simulink model "board_testa"  (R2021b)
settings: Solver=FixedStepAuto  StartTime=0.0  StopTime=inf  RelTol=1e-3  EnableMultiTasking=on
undefined symbols (not defined in the file or in its folder): CR, LF
libraries: arduinolib x5, embeddedblockslib x1
settings Model: ExtModeTrigDuration=2  Creator=eduar  LastModifiedBy=ernesto
settings OptimizationCC: EnhancedBackFolding=on  PassReuseOutputArgsAs=Individual arguments  ZeroExternalMemoryAtStartup=off  ZeroInternalMemoryAtStartup=off  MaxStackSize=64  OptimizeBlockOrder=speed  DifferentSizesBufferReuse=on  OptimizationCustomize=off  EfficientTunableParamExpr=on
settings DebuggingCC: ParameterTunabilityLossMsg=error
settings HardwareCC: ProdBitPerPointer=32  ProdBitPerSizeT=32  ProdBitPerPtrDiffT=32  ProdLargestAtomicInteger=Long  ProdLargestAtomicFloat=Double  ProdWordSize=32  ProdHWDeviceType=ARM Compatible->ARM Cortex  UseEmbeddedCoderFeatures=off
settings SFSimCC: SimCustomHeaderCode="#include \"script\\callback.h\""  SimUserSources=script\callback.c  MATLABDynamicMemAlloc=off
settings RTWCC: Description=Embedded Coder  SystemTargetFile=ert.tlc  HardwareBoard=Arduino Due  TemplateMakefile=ert_default_tmf  RTWUseSimCustomCode=on  CustomHeaderCode="#include \"script\\callback.h\""  CustomSource=script\callback.c  Toolchain=Arduino ARM  BuildConfiguration=Faster Runs
settings CodeAppCC: ForceParamTrailComments=on  IgnoreCustomStorageClasses=off  OperatorAnnotations=on  SimulinkDataObjDesc=on  SFDataObjDesc=on  InsertBlockDesc=on
settings ERTTargetCC: SupportContinuousTime=on  SupportNonInlinedSFcns=on  SupportVariableSizeSignals=on  ExtModeTransport=3  ExtModeStaticAlloc=on  ExtModeStaticAllocSize=24576  ExtModeMexFile=ext_xcp  ExtModeIntrfLevel=Level2 - Open

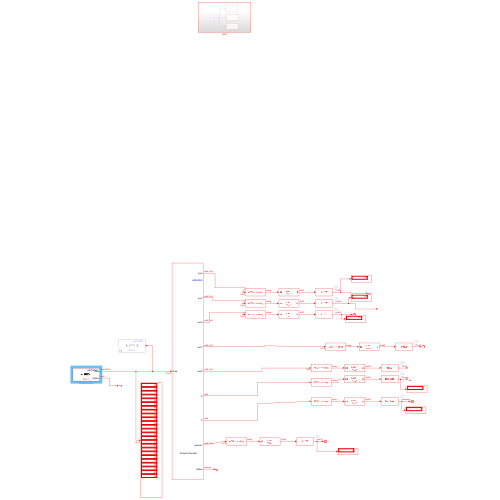
[thumbnail: Simulink's stored preview of the top-level diagram]
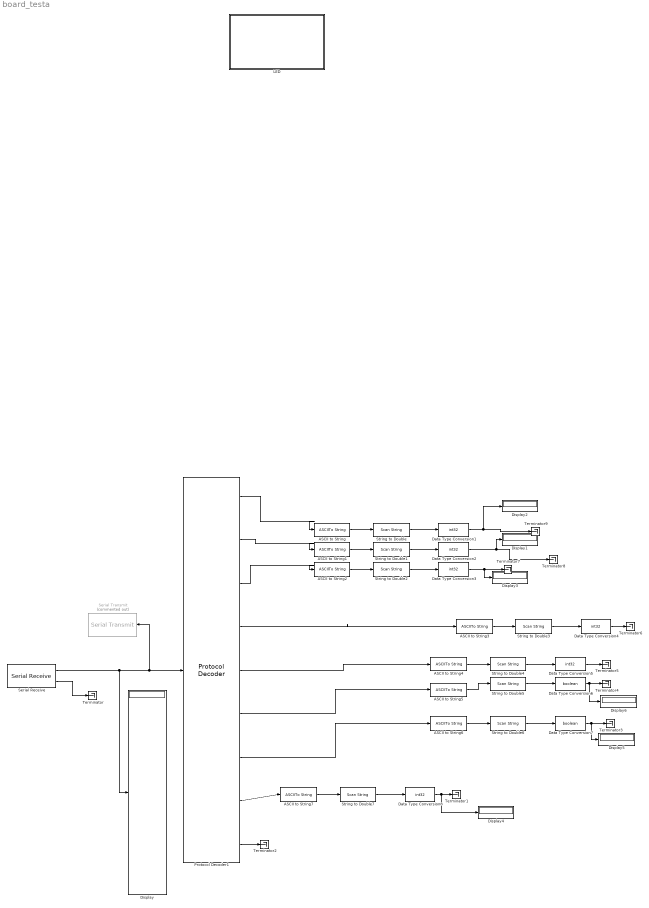
== system board_testa ==
  ASCII to String{,1..7} (8 alike) : ASCIIToString
  Data Type Conversion{1..5,8} (6 alike) : DataTypeConversion  OutDataTypeStr=int32  RndMeth=Round
  Data Type Conversion6 : DataTypeConversion  OutDataTypeStr=boolean  RndMeth=Round
  Data Type Conversion7 : DataTypeConversion  OutDataTypeStr=boolean  RndMeth=Round
  Display{,1..6} (7 alike) : Display
  LED : Subsystem
  Protocol Decoder1 : embeddedblockslib/Protocol Decoder  IsParseCSV=off  Header='@'  FieldTable={ 'joyX', '4', 'uint8', 'Little endian'; 'joyY', '4', 'uint8', 'Little endian'; 'accX', '4', 'uint8', 'Little endian'; 'accY', '4', 'uint8', 'Little endian'; 'accZ', '4', 'uint8', 'Little endian'; 'Z', '1', 'uint8', 'Little endian'; 'C', '1', 'uint8', 'Little endian'; 'remote1', '2', 'uint8', 'Little endian' }  IsVariableSizeLastField=off  MaxVariableSizeFieldLength=[]  IsChecksumRequired=off  ChecksumAlgorithm=XOR of bytes  ChecksumSize=[]  TerminatorOption=CR/LF ('\r\n')  CustomTerminatorVal=[]  IsInputLengthAvailable=off  Logo=ARDUINO
      settings: SourceProductBaseCode=ARDUINO,TIC2000
  Serial Receive : arduinolib/Serial Receive  isARMArch=on  portNumber=1  DataType=uint8  Datalength=25  SampleTime=0.01  showOutStatus=on  blockPlatform=arduino
      settings: SourceProductBaseCode=ARDUINO
  Serial Transmit : arduinolib/Serial Transmit  Commented=on  portNumber=0  sendmode=write  sendformat=Decimal  floatprecision=2  blockPlatform=arduino
  String to Double : ScanString  Format="\"%d\""
  String to Double1 : ScanString  Format="\"%d\""
  String to Double2 : ScanString  Format="\"%d\""
  String to Double{3..7} (5 alike) : ScanString  Format="\"%u\""
  Terminator{,1..9} (10 alike) : Terminator
  wires:
  String to Double2/1 -> Data Type Conversion3/1
  String to Double1/1 -> Data Type Conversion2/1
  ASCII to String2/1 -> String to Double2/1
  Protocol Decoder1/1 -> ASCII to String/1
  ASCII to String/1 -> String to Double/1
  String to Double/1 -> Data Type Conversion1/1
  Protocol Decoder1/2 -> ASCII to String1/1
  Protocol Decoder1/3 -> ASCII to String2/1
  ASCII to String1/1 -> String to Double1/1
  Serial Receive/2 -> Terminator/1
  Serial Receive/1 -> Serial Transmit/1, Protocol Decoder1/1, Display/1
  Protocol Decoder1/9 -> Terminator2/1
  ASCII to String4/1 -> String to Double4/1
  Protocol Decoder1/5 -> ASCII to String4/1
  String to Double3/1 -> Data Type Conversion4/1
  ASCII to String5/1 -> String to Double5/1
  Protocol Decoder1/6 -> ASCII to String5/1
  Protocol Decoder1/4 -> ASCII to String3/1
  String to Double4/1 -> Data Type Conversion5/1
  String to Double5/1 -> Data Type Conversion6/1
  ASCII to String3/1 -> String to Double3/1
  ASCII to String6/1 -> String to Double6/1
  String to Double6/1 -> Data Type Conversion7/1
  Protocol Decoder1/7 -> ASCII to String6/1
  ASCII to String7/1 -> String to Double7/1
  String to Double7/1 -> Data Type Conversion8/1
  Protocol Decoder1/8 -> ASCII to String7/1
  Data Type Conversion8/1 -> Display4/1, Terminator1/1
  Data Type Conversion7/1 -> Display5/1, Terminator3/1
  Data Type Conversion6/1 -> Display6/1, Terminator4/1
  Data Type Conversion5/1 -> Terminator5/1
  Data Type Conversion4/1 -> Terminator6/1
  Data Type Conversion3/1 -> Display3/1, Terminator7/1
  Data Type Conversion2/1 -> Display1/1, Terminator8/1
  Data Type Conversion1/1 -> Display2/1, Terminator9/1

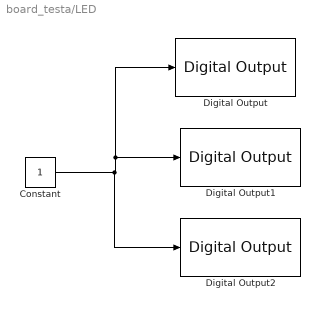
== system board_testa/LED ==
  Constant : Constant
  Digital Output : arduinolib/Digital Output  pinNumber=47  Direction=output  blockPlatform=arduino
  Digital Output1 : arduinolib/Digital Output  pinNumber=45  Direction=output  blockPlatform=arduino
  Digital Output2 : arduinolib/Digital Output  pinNumber=43  Direction=output  blockPlatform=arduino
  wires:
  Constant/1 -> Digital Output2/1, Digital Output1/1, Digital Output/1
